simulink model "TestingWatch"  (R2022b)
settings: Solver=VariableStepAuto  StartTime=0.0  StopTime=inf  RelTol=1e-3
settings Model: Creator=JJAME171  LastModifiedBy=JJAME171

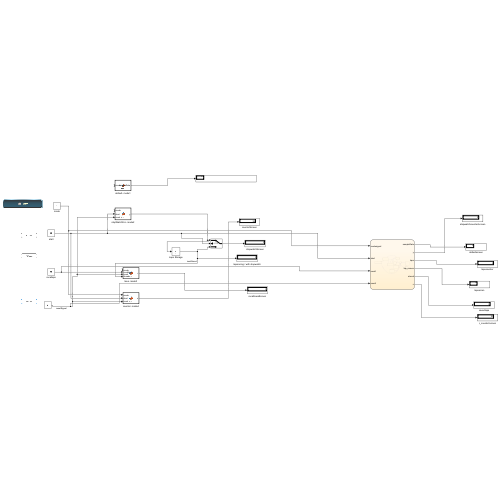
[thumbnail: Simulink's stored preview of the top-level diagram]
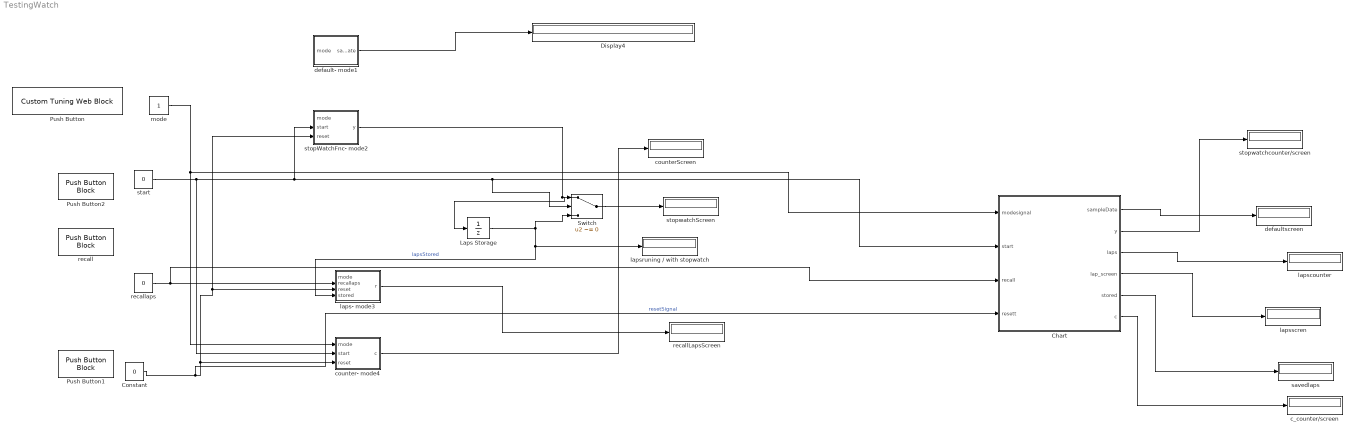
== system TestingWatch ==
  Chart : Stateflow chart  TreatAsAtomicUnit=on
  Constant : Constant  Value=0
  Display4 : Display
  Laps Storage : UnitDelay  SampleTime=-1  HasFrameUpgradeWarning=on
  Push Button : CustomTuningWebBlock  LabelPosition=Hide  ShowInitialText=on  Configuration="{\"components\":[{\"name\":\"BackgroundImageComponent\",\"settings\":{\"image\":{\"size\":[0,0],\"src\":\"default\",\"srcOrientation\":\"horizontal\"},\"position\":[0,0,1,1],\"scaleMode\":\"0\"}},{\"name\":\"ButtonStateComponent\",\"settings\":{\"buttonType\":\"latch\",\"clickFcn\":\"\",\"image\":{\"size\":[180,45],\"srcOrientation\":\"Right\"},\"latched\":false,\"offValue\":null,\"onValue\":1,\"position\":[0,0,1,1],\"pressDelay\":\"0\",\"pressFcn\":\"increment_constant\",\"repeatInterval\":\"0\",\"states\":[{\"horizontalAlignment\":\"center\",\"image\":{\"position\":[0.04444444444444445,0.005555555555555536,0.9888888888888889,0.9111111111111111],\"size\":[0.9888888888888889,0.9111111111111111],\"src\":\"data:image\\/svg+xml;base64,PHN2ZyB4bWxucz0iaHR0cDovL3d3dy53My5vcmcvMjAwMC9zdmciIHhtbG5zOnhsaW5rPSJodHRwOi8vd3d3LnczLm9yZy8xOTk5L3hsaW5rIiB2aWV3Qm94PSIwIDAgMTc3LjI1IDQwLjg4Ij48ZGVmcz48c3R5bGU+LmNscy0xe2ZpbGw6dXJsKCNyYWRpYWwtZ3JhZGllbnQpO30uY2xzLTJ7ZmlsbDp1cmwoI2xpbmVhci1ncmFkaWVudCk7fS5jbHMtM3tmaWxsOnVybCgjbGluZWFyLWdyYWRpZW50LTIpO308L3N0eWxlPjxyYWRpYWxHcmFkaWVudCBpZD0icmFkaWFsLWdyYWRpZW50IiBjeD0iOTAuMDkiIGN5PSIyMi42NiIgcj0i ...(+2212 chars)\",\"srcOrientation\":\"Right\"},\"label\":{\"color\":[1,1,0.78,1],\"icon\":{\"size\":[0.1,0.375],\"src\":\"data:image\\/svg+xml;base64,PHN2ZyBpZD0iT2ZmIiB4bWxucz0iaHR0cDovL3d3dy53My5vcmcvMjAwMC9zdmciIHhtbG5zOnhsaW5rPSJodHRwOi8vd3d3LnczLm9yZy8xOTk5L3hsaW5rIiB2aWV3Qm94PSIwIDAgNTAgNTAiPjxkZWZzPjxzdHlsZT4uY2xzLTF7ZmlsbDojN2Y4MDgwO3N0cm9rZTojMjcyNjI2O3N0cm9rZS1taXRlcmxpbWl0OjEwO3N0cm9rZS13aWR0aDozcHg7fS5jbHMtMntmaWxsOnVybCgjbGluZWFyLWdyYWRpZW50KTt9PC9zdHlsZT48bGluZWFyR3JhZGllbnQgaWQ9ImxpbmVhci1ncmFkaWVudCIgeDE9IjI1IiB5MT0iOSIgeDI9IjI1IiB5Mj0iMzciIGdyYWRpZW50VW5pdHM9InVzZXJTcGFjZU9uVXNlIj48c3RvcCBvZmZzZXQ9IjAiIHN0b3AtY29sb3I9IiNmZmYiIHN0b3Atb3BhY2l0eT0iMC43NSIvPjxzdG9wIG9mZnNldD0iMSIgc3RvcC1jb2xvcj0iI2ZmZiIgc3RvcC1vcGFjaXR5PSIwIi8+PC9saW5lYXJHcmFkaWVudD48L2RlZnM+PGNpcmNsZSBjbGFzcz0iY2xzLTEiIGN4PSIyNSIgY3k9IjI1IiByPSIyMCIvPjxjaXJjbGUgY2xhc3M9ImNscy0yIiBjeD0iMjUiIGN5PSIyMyIgcj0iMTQiLz48L3N2Zz4=\",\"srcOrientation\":\"Right\"},\"iconPlacement\":\"left\",\"opacity\":1,\"show\":true,\"text\":{\"content\":\"Button\",\"font\":\"Helvetica\",\"fontSize\":8.75}},\"labelOffset\":[0,0],\"verticalAlignment\":\"middle\"},{\"horizontalAlignment\":\"center\",\"image\":{\"position\":[0.04444444444444445,0.005555555555555536,0.9888888888888889,0.9111111111111111],\"size\":[0.9888888888888889,0.9111111111111111],\"src\":\"data:image\\/svg+xml;base64,PHN2ZyB4bWxucz0iaHR0cDovL3d3dy53My5vcmcvMjAwMC9zdmciIHhtbG5zOnhsaW5rPSJodHRwOi8vd3d3LnczLm9yZy8xOTk5L3hsaW5rIiB2aWV3Qm94PSIwIDAgMTc3LjI1IDQwLjg4Ij48ZGVmcz48c3R5bGU+LmNscy0xe2ZpbGw6dXJsKCNyYWRpYWwtZ3JhZGllbnQpO30uY2xzLTJ7ZmlsbDp1cmwoI2xpbmVhci1ncmFkaWVudCk7fS5jbHMtM3tmaWxsOnVybCgjbGluZWFyLWdyYWRpZW50LTIpO308L3N0eWxlPjxyYWRpYWxHcmFkaWVudCBpZD0icmFkaWFsLWdyYWRpZW50IiBjeD0iOTAuMDkiIGN5PSIyMi42NiIgcj0i ...(+2216 chars)\",\"srcOrientation\":\"Right\"},\"label\":{\"color\":[1,1,0.78,1],\"icon\":{\"size\":[0.1,0.375],\"src\":\"data:image\\/svg+xml;base64,PHN2ZyB4bWxucz0iaHR0cDovL3d3dy53My5vcmcvMjAwMC9zdmciIHhtbG5zOnhsaW5rPSJodHRwOi8vd3d3LnczLm9yZy8xOTk5L3hsaW5rIiB2aWV3Qm94PSIwIDAgNTAgNTAiPjxkZWZzPjxzdHlsZT4uY2xzLTF7ZmlsbDojNmFiZDQ1O3N0cm9rZTojMjcyNjI2O3N0cm9rZS1taXRlcmxpbWl0OjEwO3N0cm9rZS13aWR0aDozcHg7fS5jbHMtMntmaWxsOnVybCgjbGluZWFyLWdyYWRpZW50KTt9PC9zdHlsZT48bGluZWFyR3JhZGllbnQgaWQ9ImxpbmVhci1ncmFkaWVudCIgeDE9IjI1IiB5MT0iOSIgeDI9IjI1IiB5Mj0iMzciIGdyYWRpZW50VW5pdHM9InVzZXJTcGFjZU9uVXNlIj48c3RvcCBvZmZzZXQ9IjAiIHN0b3AtY29sb3I9IiNmZmYiIHN0b3Atb3BhY2l0eT0iMC43NSIvPjxzdG9wIG9mZnNldD0iMSIgc3RvcC1jb2xvcj0iI2ZmZiIgc3RvcC1vcGFjaXR5PSIwIi8+PC9saW5lYXJHcmFkaWVudD48L2RlZnM+PGcgaWQ9Ik9uIj48Y2lyY2xlIGNsYXNzPSJjbHMtMSIgY3g9IjI1IiBjeT0iMjUiIHI9IjIwIi8+PGNpcmNsZSBjbGFzcz0iY2xzLTIiIGN4PSIyNSIgY3k9IjIzIiByPSIxNCIvPjwvZz48L3N2Zz4=\",\"srcOrientation\":\"Right\"},\"iconPlacement\":\"left\",\"opacity\":1,\"show\":true,\"text\":{\"content\":\"Button\",\"font\":\"Helvetica\",\"fontSize\":8.75}},\"labelOffset\":[0.025,0],\"verticalAlignment\":\"middle\"},{\"horizontalAlignment\":\"center\",\"image\":{\"position\":[0.04444444444444445,0.005555555555555536,0.9888888888888889,0.9111111111111111],\"size\":[0.9888888888888889,0.9111111111111111],\"src\":\"data:image\\/svg+xml;base64,PHN2ZyB4bWxucz0iaHR0cDovL3d3dy53My5vcmcvMjAwMC9zdmciIHhtbG5zOnhsaW5rPSJodHRwOi8vd3d3LnczLm9yZy8xOTk5L3hsaW5rIiB2aWV3Qm94PSIwIDAgMTc3LjI1IDQwLjg4Ij48ZGVmcz48c3R5bGU+LmNscy0xe2ZpbGw6dXJsKCNyYWRpYWwtZ3JhZGllbnQpO30uY2xzLTJ7ZmlsbDp1cmwoI2xpbmVhci1ncmFkaWVudCk7fS5jbHMtM3tmaWxsOnVybCgjbGluZWFyLWdyYWRpZW50LTIpO308L3N0eWxlPjxyYWRpYWxHcmFkaWVudCBpZD0icmFkaWFsLWdyYWRpZW50IiBjeD0iOTAuMDkiIGN5PSIyMi42NiIgcj0i ...(+2212 chars)\",\"srcOrientation\":\"Right\"},\"label\":{\"color\":[1,1,0.78,1],\"icon\":{\"size\":[0.1,0.375],\"src\":\"data:image\\/svg+xml;base64,PHN2ZyB4bWxucz0iaHR0cDovL3d3dy53My5vcmcvMjAwMC9zdmciIHhtbG5zOnhsaW5rPSJodHRwOi8vd3d3LnczLm9yZy8xOTk5L3hsaW5rIiB2aWV3Qm94PSIwIDAgNTAgNTAiPjxkZWZzPjxzdHlsZT4uY2xzLTF7ZmlsbDojNmFiZDQ1O3N0cm9rZTojMjcyNjI2O3N0cm9rZS1taXRlcmxpbWl0OjEwO3N0cm9rZS13aWR0aDozcHg7fS5jbHMtMntmaWxsOnVybCgjbGluZWFyLWdyYWRpZW50KTt9PC9zdHlsZT48bGluZWFyR3JhZGllbnQgaWQ9ImxpbmVhci1ncmFkaWVudCIgeDE9IjI1IiB5MT0iOSIgeDI9IjI1IiB5Mj0iMzciIGdyYWRpZW50VW5pdHM9InVzZXJTcGFjZU9uVXNlIj48c3RvcCBvZmZzZXQ9IjAiIHN0b3AtY29sb3I9IiNmZmYiIHN0b3Atb3BhY2l0eT0iMC43NSIvPjxzdG9wIG9mZnNldD0iMSIgc3RvcC1jb2xvcj0iI2ZmZiIgc3RvcC1vcGFjaXR5PSIwIi8+PC9saW5lYXJHcmFkaWVudD48L2RlZnM+PGcgaWQ9Ik9uIj48Y2lyY2xlIGNsYXNzPSJjbHMtMSIgY3g9IjI1IiBjeT0iMjUiIHI9IjIwIi8+PGNpcmNsZSBjbGFzcz0iY2xzLTIiIGN4PSIyNSIgY3k9IjIzIiByPSIxNCIvPjwvZz48L3N2Zz4=\",\"srcOrientation\":\"Right\"},\"iconPlacement\":\"left\",\"opacity\":1,\"show\":true,\"text\":{\"content\":\"Button\",\"font\":\"Helvetica\",\"fontSize\":8.75}},\"labelOffset\":[0,0],\"verticalAlignment\":\"middle\"},{\"horizontalAlignment\":\"center\",\"image\":{\"position\":[0.04444444444444445,0.005555555555555536,0.9888888888888889,0.9111111111111111],\"size\":[0.9888888888888889,0.9111111111111111],\"src\":\"data:image\\/svg+xml;base64,PHN2ZyB4bWxucz0iaHR0cDovL3d3dy53My5vcmcvMjAwMC9zdmciIHhtbG5zOnhsaW5rPSJodHRwOi8vd3d3LnczLm9yZy8xOTk5L3hsaW5rIiB2aWV3Qm94PSIwIDAgMTc3LjI1IDQwLjg4Ij48ZGVmcz48c3R5bGU+LmNscy0xe2ZpbGw6dXJsKCNyYWRpYWwtZ3JhZGllbnQpO30uY2xzLTJ7ZmlsbDp1cmwoI2xpbmVhci1ncmFkaWVudCk7fS5jbHMtM3tmaWxsOnVybCgjbGluZWFyLWdyYWRpZW50LTIpO308L3N0eWxlPjxyYWRpYWxHcmFkaWVudCBpZD0icmFkaWFsLWdyYWRpZW50IiBjeD0iOTAuMDkiIGN5PSIyMi42NiIgcj0i ...(+2216 chars)\",\"srcOrientation\":\"Right\"},\"label\":{\"color\":[1,1,0.78,1],\"icon\":{\"size\":[0.1,0.375],\"src\":\"data:image\\/svg+xml;base64,PHN2ZyBpZD0iT2ZmIiB4bWxucz0iaHR0cDovL3d3dy53My5vcmcvMjAwMC9zdmciIHhtbG5zOnhsaW5rPSJodHRwOi8vd3d3LnczLm9yZy8xOTk5L3hsaW5rIiB2aWV3Qm94PSIwIDAgNTAgNTAiPjxkZWZzPjxzdHlsZT4uY2xzLTF7ZmlsbDojN2Y4MDgwO3N0cm9rZTojMjcyNjI2O3N0cm9rZS1taXRlcmxpbWl0OjEwO3N0cm9rZS13aWR0aDozcHg7fS5jbHMtMntmaWxsOnVybCgjbGluZWFyLWdyYWRpZW50KTt9PC9zdHlsZT48bGluZWFyR3JhZGllbnQgaWQ9ImxpbmVhci1ncmFkaWVudCIgeDE9IjI1IiB5MT0iOSIgeDI9IjI1IiB5Mj0iMzciIGdyYWRpZW50VW5pdHM9InVzZXJTcGFjZU9uVXNlIj48c3RvcCBvZmZzZXQ9IjAiIHN0b3AtY29sb3I9IiNmZmYiIHN0b3Atb3BhY2l0eT0iMC43NSIvPjxzdG9wIG9mZnNldD0iMSIgc3RvcC1jb2xvcj0iI2ZmZiIgc3RvcC1vcGFjaXR5PSIwIi8+PC9saW5lYXJHcmFkaWVudD48L2RlZnM+PGNpcmNsZSBjbGFzcz0iY2xzLTEiIGN4PSIyNSIgY3k9IjI1IiByPSIyMCIvPjxjaXJjbGUgY2xhc3M9ImNscy0yIiBjeD0iMjUiIGN5PSIyMyIgcj0iMTQiLz48L3N2Zz4=\",\"srcOrientation\":\"Right\"},\"iconPlacement\":\"left\",\"opacity\":1,\"show\":true,\"text\":{\"content\":\"Button\",\"font\":\"Helvetica\",\"fontSize\":8.75}},\"labelOffset\":[0.025,0],\"verticalAlignment\":\"middle\"}]}},{\"name\":\"ForegroundImageComponent\",\"settings\":{\"image\":{\"size\":[0,0],\"src\":\"default\",\"srcOrientation\":\"horizontal\"},\"isForeground\":1,\"position\":[0,0,1,1],\"scaleMode\":\"0\"}}],\"settings\":{\"BindingType\":\"param\",\"aspectRatio\":3.7777777777777777,\"backgroundColor\":[0,0,0,\"1\"],\"backgroundOffset\":0,\"backgroundOpacity\":1,\"fixedAspectRatio\":\"off\",\"foregroundColor\":[252,252,196],\"showBackgroundColor\":false,\"variant\":\"push\",\"version\":\"22b\"},\"type\":\"Button\"}"
  Push Button1 : PushButtonBlock  ButtonText=RESET  ButtonType=Latch  IconColor=On  OffValue=0.000000
  Push Button2 : PushButtonBlock  ButtonText=START  ButtonType=Latch  IconColor=On  OffValue=0.000000
  Switch : Switch  Criteria=u2 ~= 0  Threshold=1  SaturateOnIntegerOverflow=off  InputSameDT=off
  c_counter/screen : Display
  counter- mode4 : MATLAB Function  TreatAsAtomicUnit=on
  counterScreen : Display
  default- mode1 : MATLAB Function  TreatAsAtomicUnit=on
  defaultscreen : Display
  laps- mode3 : MATLAB Function  TreatAsAtomicUnit=on
  lapscounter : Display
  lapsruning / with stopwatch : Display
  lapsscren : Display
  mode : Constant  OutDataTypeStr=double
  recall : PushButtonBlock  ButtonText=RECALL  ButtonType=Latch  IconColor=On  OffValue=0.000000
  recallLapsScreen : Display
  recallaps : Constant  Value=0  OutDataTypeStr=double
  savedlaps : Display
  start : Constant  Value=0  OutDataTypeStr=double
  stopWatchFnc- mode2 : MATLAB Function  TreatAsAtomicUnit=on
  stopwatchScreen : Display
  stopwatchcounter/screen : Display
  wires:
  mode/1 -> Chart/1(modesignal), counter- mode4/1(mode)
  start/1 -> Chart/2(start), Switch/2, stopWatchFnc- mode2/2(start), counter- mode4/2(start)
  stopWatchFnc- mode2/1(y) -> Laps Storage/1, Switch/1
  Switch/1 -> stopwatchScreen/1
  recallaps/1 -> Chart/3(recall), laps- mode3/2(recallaps)
  Laps Storage/1 -> lapsruning / with stopwatch/1, laps- mode3/4(stored), Switch/3  "lapsStored"
  Constant/1 -> Chart/4(resett), laps- mode3/3(reset), stopWatchFnc- mode2/3(reset), counter- mode4/3(reset)  "resetSignal"
  laps- mode3/1(r) -> recallLapsScreen/1
  counter- mode4/1(c) -> counterScreen/1
  default- mode1/1(sampleDate) -> Display4/1
  Chart/2(y) -> stopwatchcounter/screen/1
  Chart/1(sampleDate) -> defaultscreen/1
  Chart/3(laps) -> lapscounter/1
  Chart/4(lap_screen) -> lapsscren/1
  Chart/5(stored) -> savedlaps/1
  Chart/6(c) -> c_counter/screen/1

== matlab function TestingWatch/laps- mode3 ==
  data: mode input; r output; recallaps input; reset input; stored input


function r  = fcn(mode, recallaps, reset, stored)
   
 % Reset x if 'reset' is 1 and 'start' is 0
  if reset == 1 && recallaps == 1 && mode==3
    r = 0;

    return; % Exit early after reset

  elseif  recallaps == 1 && mode==3
      r= stored;
  else
      r=0;
  end
end

== matlab function TestingWatch/counter- mode4 ==
  data: mode input; c output; start input; reset input
function c = fcn(mode, start, reset)
  persistent counter;

  % Initialize counter if it's empty
  if isempty(counter)
    counter = 30;
  end

  % Reset the counter if 'reset' is 1, 'start' is 0 and 'mode' is 3
  if reset == 1 && start == 0 && mode==4
    counter = 30;
    c = 30;
    return; % Exit early after reset
  else
      c=counter;
  end

  % Decrement counter based on 'mode', 'start' and counter
  if start == 1
    if mode == 4 &&  counter>=1
        %c = counter;
      counter = counter - 1;
    end
    
  elseif start == 0
    c = counter; % Return current counter value
  else
    c = 30; % Handle invalid 'start' values
  end
end

== matlab function TestingWatch/default- mode1 ==
  data: mode input; sampleDate output string
function sampleDate = fcn(mode)
if mode==1
    sampleDate= "October 28 2024. 10:11am. Monday ";
else
    sampleDate= " ";
end
end

== matlab function TestingWatch/stopWatchFnc- mode2 ==
  data: mode input; y output; start input; reset input
function y = fcn(mode, start, reset)
  persistent counter;

  % Initialize counter if it's empty
  if isempty(counter)
    counter = 0;
  end

  % Reset the counter if 'reset' is 1 and 'start' is 0
  if reset == 1 && start == 0 && mode==2
    counter = 0;
    y = 0;
    return; % Exit early after reset
  end

  % Increment counter based on 'mode' and 'start'
  if start == 1
    if mode == 2
      counter = counter + 1;
    end
    y = counter;
  elseif start == 0
    y = counter; % Return current counter value
  else
    y = 0; % Handle invalid 'start' values
  end
end

== stateflow chart TestingWatch/Chart ==
  state Stopwatcht
    counter = 0;
    y= counter
  state StopwatchStop
    entry:
    laps=y
    y=laps
  state Default
    entry:
    sampleDate= "October 28 2024. 10:11am. Monday ";
    exit:
    sampleDate=""
  state CounterStart
    entry:
    counter_c=30;
    during:
    if counter_c >1
    c= counter_c
    counter_c = counter_c -1;
    end
    exit:
    c= counter_c
  state LapStorage
    entry:
    lap_screen= "LAPS"
    exit:
    lap_screen=""
    laps=y;
  state Counter
    entry:
    counter_c=30;
    c = counter_c
  state StopwatchStart
    entry:
    counter = 0;
    during:
    y= counter
    laps= y
    counter = counter + 1;
    exit:
    laps= y
  state LapStorageRecall
    entry:
    lap_screen= "LAPS"
    stored=laps
  state CounterStop
    entry:
    c= counter_c
  state LapStorageRecallReset
    entry:
    lap_screen= "LAPS"
    stored=0;
  StopwatchStop -> Stopwatcht [order 1] : [start==0 && modesignal==2&&resett==1]
  StopwatchStop -> StopwatchStart [order 3] : [start==1 && modesignal==2]
  StopwatchStart -> StopwatchStop [order 2] : [start==0 && modesignal==2]{laps=y}
  StopwatchStop -> LapStorage [order 2] : [modesignal==2 && start==0]
  Stopwatcht -> LapStorage [order 2] : [modesignal==4]
  Default -> Stopwatcht : [modesignal==2]
  Stopwatcht -> StopwatchStart [order 1] : [start==1 && modesignal==2]
  (default) -> Default
  Counter -> CounterStart [order 2] : [modesignal==4 &&start==1]
  StopwatchStart -> LapStorage [order 1] : [modesignal==3]{laps=y}
  LapStorage -> Counter [order 1] : [modesignal==4 ]
  Counter -> Default [order 1] : [modesignal==1]
  LapStorageRecallReset -> Counter : [modesignal==4]
  LapStorageRecall -> Counter [order 2] : [modesignal==4 &&recall==0]
  CounterStop -> Counter [order 2] : [modesignal==4&&start==0&&resett==1]
  LapStorage -> LapStorageRecall [order 2] : [modesignal==3&&recall==1]{laps=y}
  CounterStop -> CounterStart [order 1] : [modesignal==4 && start==1]
  CounterStart -> CounterStop : [modesignal==4 &&start==0]
  LapStorageRecall -> LapStorageRecallReset [order 1] : [modesignal==3 && recall==1 && resett==1]
  data: sampleDate output; modesignal input; start input; counter local; y output; laps output; lap_screen output string; recall input; stored output; counter_c local; c output; resett input
